simulink model "TST_EnvP_VD"  (R2016b)
settings: Solver=FixedStepDiscrete  StartTime=0.0  StopTime=simTime  FixedStep=sampleTime  RelTol=1e-3
values from neighbouring files (symbols this model uses):
  testCase = 1    [initTST_EnvP_VD_001.m]    (also in initTST_EnvP_VD_002.m = 2; initTST_EnvP_VD_003.m = 3)
libraries: simulink x7, UnitTest_Lib x3
settings Model: Creator=liangyunbo  LastModifiedBy=liangyunbo
settings DebuggingCC: SignalRangeChecking=error

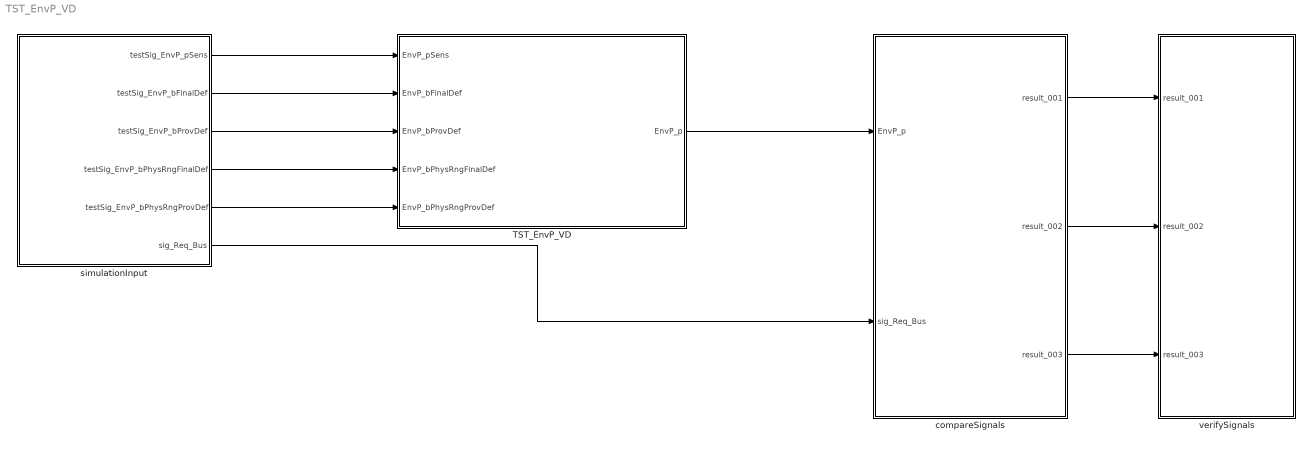
== system TST_EnvP_VD ==
  TST_EnvP_VD : Subsystem
  compareSignals : Subsystem
  simulationInput : Subsystem
  verifySignals : Subsystem
  wires:
  simulationInput/1(testSig_EnvP_pSens) -> TST_EnvP_VD/1(EnvP_pSens)
  simulationInput/2(testSig_EnvP_bFinalDef) -> TST_EnvP_VD/2(EnvP_bFinalDef)
  simulationInput/3(testSig_EnvP_bProvDef) -> TST_EnvP_VD/3(EnvP_bProvDef)
  simulationInput/4(testSig_EnvP_bPhysRngFinalDef) -> TST_EnvP_VD/4(EnvP_bPhysRngFinalDef)
  simulationInput/5(testSig_EnvP_bPhysRngProvDef) -> TST_EnvP_VD/5(EnvP_bPhysRngProvDef)
  TST_EnvP_VD/1(EnvP_p) -> compareSignals/1(EnvP_p)
  simulationInput/6(sig_Req_Bus) -> compareSignals/2(sig_Req_Bus)
  compareSignals/1(result_001) -> verifySignals/1(result_001)
  compareSignals/2(result_002) -> verifySignals/2(result_002)
  compareSignals/3(result_003) -> verifySignals/3(result_003)

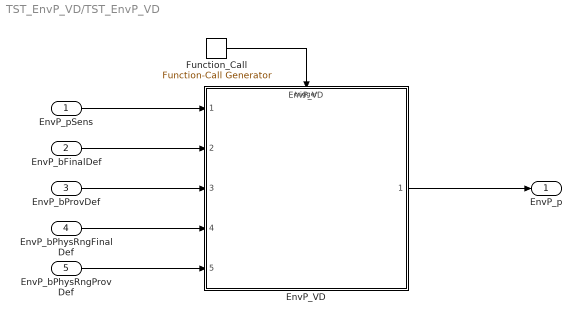
== system TST_EnvP_VD/TST_EnvP_VD ==
  EnvP_pSens : Inport
  EnvP_bFinalDef : Inport  Port=2
  EnvP_bProvDef : Inport  Port=3
  EnvP_bPhysRngFinalDef : Inport  Port=4
  EnvP_bPhysRngProvDef : Inport  Port=5
  EnvP_VD : ModelReference  ModelNameDialog=EnvP_VD  SimulationMode=Normal  ModelReferenceVersion=1.7  TriggerPortName=function  TriggerPortTriggerType=function-call  TriggerPortStatesWhenEnabling=held
  Function_Call : simulink/Ports & Subsystems/Function-Call Generator  sample_time=sampleTime  numberOfIterations=1
  EnvP_p : Outport
  wires:
  Function_Call/1 -> EnvP_VD/Trigger
  EnvP_pSens/1 -> EnvP_VD/1
  EnvP_bFinalDef/1 -> EnvP_VD/2
  EnvP_bProvDef/1 -> EnvP_VD/3
  EnvP_bPhysRngFinalDef/1 -> EnvP_VD/4
  EnvP_bPhysRngProvDef/1 -> EnvP_VD/5
  EnvP_VD/1 -> EnvP_p/1

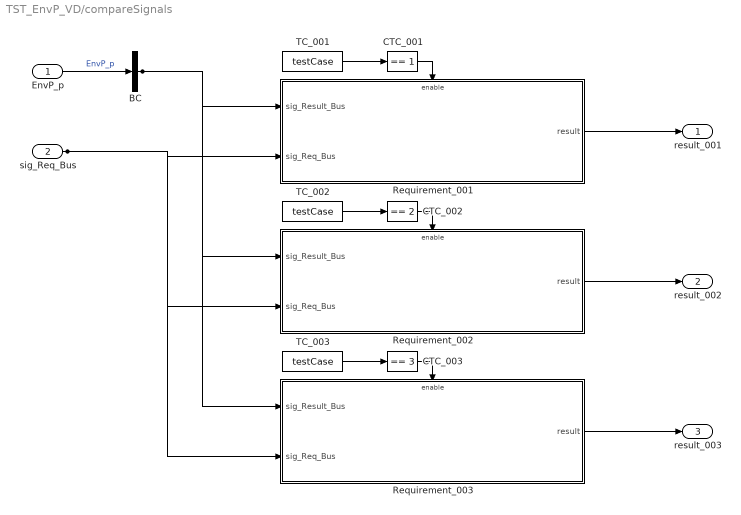
== system TST_EnvP_VD/compareSignals ==
  EnvP_p : Inport
  sig_Req_Bus : Inport  Port=2
  BC : BusCreator  Inputs=1
  CTC_001 : simulink/Logic and Bit Operations/Compare To Constant  relop===  const=1  OutDataTypeStr=boolean
  CTC_002 : simulink/Logic and Bit Operations/Compare To Constant  relop===  const=2  OutDataTypeStr=boolean
  CTC_003 : simulink/Logic and Bit Operations/Compare To Constant  relop===  const=3  OutDataTypeStr=boolean
  Requirement_001 : Subsystem
  Requirement_002 : Subsystem
  Requirement_003 : Subsystem
  TC_001 : Constant  Value=testCase
  TC_002 : Constant  Value=testCase
  TC_003 : Constant  Value=testCase
  result_001 : Outport
  result_002 : Outport  Port=2
  result_003 : Outport  Port=3
  wires:
  EnvP_p/1 -> BC/1  "EnvP_p"
  TC_001/1 -> CTC_001/1
  CTC_001/1 -> Requirement_001/Enable
  sig_Req_Bus/1 -> Requirement_001/2(sig_Req_Bus), Requirement_002/2(sig_Req_Bus), Requirement_003/2(sig_Req_Bus)
  BC/1 -> Requirement_001/1(sig_Result_Bus), Requirement_002/1(sig_Result_Bus), Requirement_003/1(sig_Result_Bus)
  Requirement_001/1(result) -> result_001/1
  TC_002/1 -> CTC_002/1
  CTC_002/1 -> Requirement_002/Enable
  Requirement_002/1(result) -> result_002/1
  TC_003/1 -> CTC_003/1
  CTC_003/1 -> Requirement_003/Enable
  Requirement_003/1(result) -> result_003/1

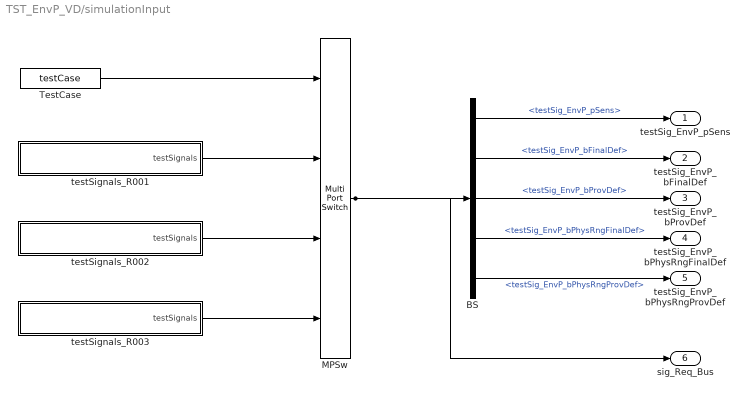
== system TST_EnvP_VD/simulationInput ==
  BS : BusSelector  OutputSignals=testSig_EnvP_pSens,testSig_EnvP_bFinalDef,testSig_EnvP_bProvDef,testSig_EnvP_bPhysRngFinalDef,testSig_EnvP_bPhysRngProvDef
  MPSw : MultiPortSwitch  SaturateOnIntegerOverflow=on  InputSameDT=on
  TestCase : Constant  Value=testCase
  testSignals_R001 : Subsystem
  testSignals_R002 : Subsystem
  testSignals_R003 : Subsystem
  testSig_EnvP_pSens : Outport
  testSig_EnvP_bFinalDef : Outport  Port=2
  testSig_EnvP_bProvDef : Outport  Port=3
  testSig_EnvP_bPhysRngFinalDef : Outport  Port=4
  testSig_EnvP_bPhysRngProvDef : Outport  Port=5
  sig_Req_Bus : Outport  Port=6
  wires:
  BS/1 -> testSig_EnvP_pSens/1  "<testSig_EnvP_pSens>"
  BS/2 -> testSig_EnvP_bFinalDef/1  "<testSig_EnvP_bFinalDef>"
  BS/3 -> testSig_EnvP_bProvDef/1  "<testSig_EnvP_bProvDef>"
  BS/4 -> testSig_EnvP_bPhysRngFinalDef/1  "<testSig_EnvP_bPhysRngFinalDef>"
  BS/5 -> testSig_EnvP_bPhysRngProvDef/1  "<testSig_EnvP_bPhysRngProvDef>"
  MPSw/1 -> BS/1, sig_Req_Bus/1
  TestCase/1 -> MPSw/1
  testSignals_R001/1(testSignals) -> MPSw/2
  testSignals_R002/1(testSignals) -> MPSw/3
  testSignals_R003/1(testSignals) -> MPSw/4

== system TST_EnvP_VD/verifySignals ==
  result_001 : Inport
  result_002 : Inport  Port=2
  result_003 : Inport  Port=3
  Assertion_001 : Assertion  Enabled=off
  Assertion_002 : Assertion  Enabled=off
  Assertion_003 : Assertion  Enabled=off
  wires:
  result_001/1 -> Assertion_001/1
  result_002/1 -> Assertion_002/1
  result_003/1 -> Assertion_003/1

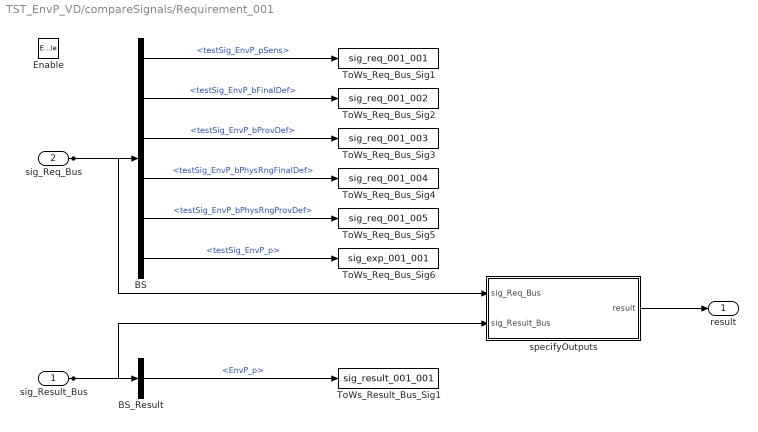
== system TST_EnvP_VD/compareSignals/Requirement_001 ==
  sig_Result_Bus : Inport
  sig_Req_Bus : Inport  Port=2
  Enable : EnablePort
  BS : BusSelector  OutputSignals=testSig_EnvP_pSens,testSig_EnvP_bFinalDef,testSig_EnvP_bProvDef,testSig_EnvP_bPhysRngFinalDef,testSig_EnvP_bPhysRngProvDef,testSig_EnvP_p
  BS_Result : BusSelector  OutputSignals=EnvP_p
  ToWs_Req_Bus_Sig1 : ToWorkspace  VariableName=sig_req_001_001  SaveFormat=Structure With Time
  ToWs_Req_Bus_Sig2 : ToWorkspace  VariableName=sig_req_001_002  SaveFormat=Structure With Time
  ToWs_Req_Bus_Sig3 : ToWorkspace  VariableName=sig_req_001_003  SaveFormat=Structure With Time
  ToWs_Req_Bus_Sig4 : ToWorkspace  VariableName=sig_req_001_004  SaveFormat=Structure With Time
  ToWs_Req_Bus_Sig5 : ToWorkspace  VariableName=sig_req_001_005  SaveFormat=Structure With Time
  ToWs_Req_Bus_Sig6 : ToWorkspace  VariableName=sig_exp_001_001  SaveFormat=Structure With Time
  ToWs_Result_Bus_Sig1 : ToWorkspace  VariableName=sig_result_001_001  SaveFormat=Structure With Time
  specifyOutputs : Subsystem
  result : Outport
  wires:
  sig_Req_Bus/1 -> BS/1, specifyOutputs/1(sig_Req_Bus)
  BS/1 -> ToWs_Req_Bus_Sig1/1  "<testSig_EnvP_pSens>"
  BS/2 -> ToWs_Req_Bus_Sig2/1  "<testSig_EnvP_bFinalDef>"
  BS/3 -> ToWs_Req_Bus_Sig3/1  "<testSig_EnvP_bProvDef>"
  BS/4 -> ToWs_Req_Bus_Sig4/1  "<testSig_EnvP_bPhysRngFinalDef>"
  BS/5 -> ToWs_Req_Bus_Sig5/1  "<testSig_EnvP_bPhysRngProvDef>"
  BS/6 -> ToWs_Req_Bus_Sig6/1  "<testSig_EnvP_p>"
  sig_Result_Bus/1 -> BS_Result/1, specifyOutputs/2(sig_Result_Bus)
  BS_Result/1 -> ToWs_Result_Bus_Sig1/1  "<EnvP_p>"
  specifyOutputs/1(result) -> result/1

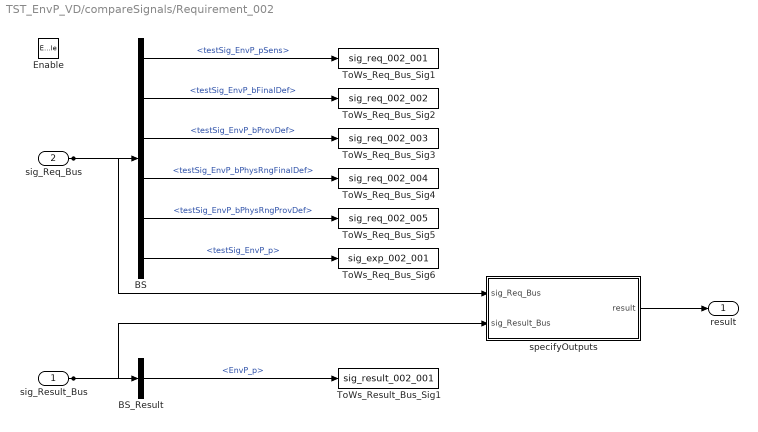
== system TST_EnvP_VD/compareSignals/Requirement_002 ==
  sig_Result_Bus : Inport
  sig_Req_Bus : Inport  Port=2
  Enable : EnablePort
  BS : BusSelector  OutputSignals=testSig_EnvP_pSens,testSig_EnvP_bFinalDef,testSig_EnvP_bProvDef,testSig_EnvP_bPhysRngFinalDef,testSig_EnvP_bPhysRngProvDef,testSig_EnvP_p
  BS_Result : BusSelector  OutputSignals=EnvP_p
  ToWs_Req_Bus_Sig1 : ToWorkspace  VariableName=sig_req_002_001  SaveFormat=Structure With Time
  ToWs_Req_Bus_Sig2 : ToWorkspace  VariableName=sig_req_002_002  SaveFormat=Structure With Time
  ToWs_Req_Bus_Sig3 : ToWorkspace  VariableName=sig_req_002_003  SaveFormat=Structure With Time
  ToWs_Req_Bus_Sig4 : ToWorkspace  VariableName=sig_req_002_004  SaveFormat=Structure With Time
  ToWs_Req_Bus_Sig5 : ToWorkspace  VariableName=sig_req_002_005  SaveFormat=Structure With Time
  ToWs_Req_Bus_Sig6 : ToWorkspace  VariableName=sig_exp_002_001  SaveFormat=Structure With Time
  ToWs_Result_Bus_Sig1 : ToWorkspace  VariableName=sig_result_002_001  SaveFormat=Structure With Time
  specifyOutputs : Subsystem
  result : Outport
  wires:
  sig_Req_Bus/1 -> BS/1, specifyOutputs/1(sig_Req_Bus)
  BS/1 -> ToWs_Req_Bus_Sig1/1  "<testSig_EnvP_pSens>"
  BS/2 -> ToWs_Req_Bus_Sig2/1  "<testSig_EnvP_bFinalDef>"
  BS/3 -> ToWs_Req_Bus_Sig3/1  "<testSig_EnvP_bProvDef>"
  BS/4 -> ToWs_Req_Bus_Sig4/1  "<testSig_EnvP_bPhysRngFinalDef>"
  BS/5 -> ToWs_Req_Bus_Sig5/1  "<testSig_EnvP_bPhysRngProvDef>"
  BS/6 -> ToWs_Req_Bus_Sig6/1  "<testSig_EnvP_p>"
  sig_Result_Bus/1 -> BS_Result/1, specifyOutputs/2(sig_Result_Bus)
  BS_Result/1 -> ToWs_Result_Bus_Sig1/1  "<EnvP_p>"
  specifyOutputs/1(result) -> result/1

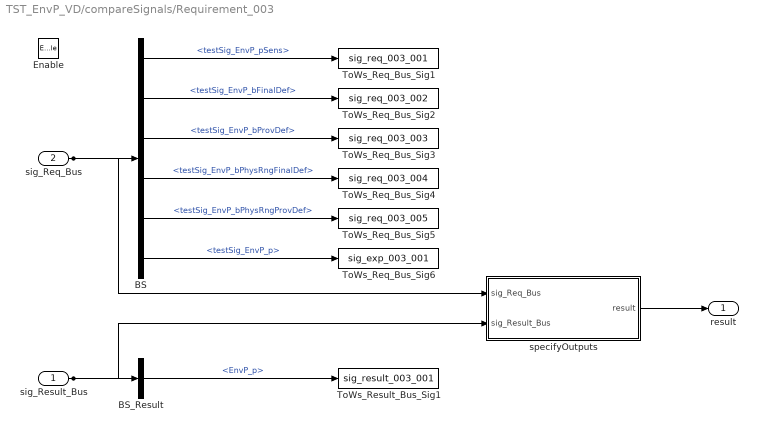
== system TST_EnvP_VD/compareSignals/Requirement_003 ==
  sig_Result_Bus : Inport
  sig_Req_Bus : Inport  Port=2
  Enable : EnablePort
  BS : BusSelector  OutputSignals=testSig_EnvP_pSens,testSig_EnvP_bFinalDef,testSig_EnvP_bProvDef,testSig_EnvP_bPhysRngFinalDef,testSig_EnvP_bPhysRngProvDef,testSig_EnvP_p
  BS_Result : BusSelector  OutputSignals=EnvP_p
  ToWs_Req_Bus_Sig1 : ToWorkspace  VariableName=sig_req_003_001  SaveFormat=Structure With Time
  ToWs_Req_Bus_Sig2 : ToWorkspace  VariableName=sig_req_003_002  SaveFormat=Structure With Time
  ToWs_Req_Bus_Sig3 : ToWorkspace  VariableName=sig_req_003_003  SaveFormat=Structure With Time
  ToWs_Req_Bus_Sig4 : ToWorkspace  VariableName=sig_req_003_004  SaveFormat=Structure With Time
  ToWs_Req_Bus_Sig5 : ToWorkspace  VariableName=sig_req_003_005  SaveFormat=Structure With Time
  ToWs_Req_Bus_Sig6 : ToWorkspace  VariableName=sig_exp_003_001  SaveFormat=Structure With Time
  ToWs_Result_Bus_Sig1 : ToWorkspace  VariableName=sig_result_003_001  SaveFormat=Structure With Time
  specifyOutputs : Subsystem
  result : Outport
  wires:
  sig_Req_Bus/1 -> BS/1, specifyOutputs/1(sig_Req_Bus)
  BS/1 -> ToWs_Req_Bus_Sig1/1  "<testSig_EnvP_pSens>"
  BS/2 -> ToWs_Req_Bus_Sig2/1  "<testSig_EnvP_bFinalDef>"
  BS/3 -> ToWs_Req_Bus_Sig3/1  "<testSig_EnvP_bProvDef>"
  BS/4 -> ToWs_Req_Bus_Sig4/1  "<testSig_EnvP_bPhysRngFinalDef>"
  BS/5 -> ToWs_Req_Bus_Sig5/1  "<testSig_EnvP_bPhysRngProvDef>"
  BS/6 -> ToWs_Req_Bus_Sig6/1  "<testSig_EnvP_p>"
  sig_Result_Bus/1 -> BS_Result/1, specifyOutputs/2(sig_Result_Bus)
  BS_Result/1 -> ToWs_Result_Bus_Sig1/1  "<EnvP_p>"
  specifyOutputs/1(result) -> result/1

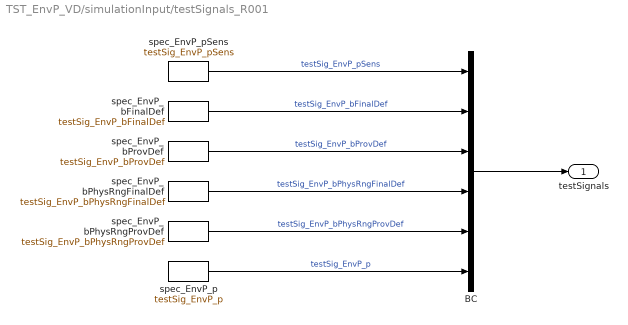
== system TST_EnvP_VD/simulationInput/testSignals_R001 ==
  BC : BusCreator  Inputs=6
  spec_EnvP_bFinalDef : FromWorkspace  VariableName=testSig_EnvP_bFinalDef  Interpolate=off  OutputAfterFinalValue=Holding final value
  spec_EnvP_bPhysRngFinalDef : FromWorkspace  VariableName=testSig_EnvP_bPhysRngFinalDef  Interpolate=off  OutputAfterFinalValue=Holding final value
  spec_EnvP_bPhysRngProvDef : FromWorkspace  VariableName=testSig_EnvP_bPhysRngProvDef  Interpolate=off  OutputAfterFinalValue=Holding final value
  spec_EnvP_bProvDef : FromWorkspace  VariableName=testSig_EnvP_bProvDef  Interpolate=off  OutputAfterFinalValue=Holding final value
  spec_EnvP_p : FromWorkspace  VariableName=testSig_EnvP_p  Interpolate=off  OutputAfterFinalValue=Holding final value
  spec_EnvP_pSens : FromWorkspace  VariableName=testSig_EnvP_pSens  Interpolate=off  OutputAfterFinalValue=Holding final value
  testSignals : Outport
  wires:
  BC/1 -> testSignals/1
  spec_EnvP_pSens/1 -> BC/1  "testSig_EnvP_pSens"
  spec_EnvP_bFinalDef/1 -> BC/2  "testSig_EnvP_bFinalDef"
  spec_EnvP_bProvDef/1 -> BC/3  "testSig_EnvP_bProvDef"
  spec_EnvP_bPhysRngFinalDef/1 -> BC/4  "testSig_EnvP_bPhysRngFinalDef"
  spec_EnvP_bPhysRngProvDef/1 -> BC/5  "testSig_EnvP_bPhysRngProvDef"
  spec_EnvP_p/1 -> BC/6  "testSig_EnvP_p"

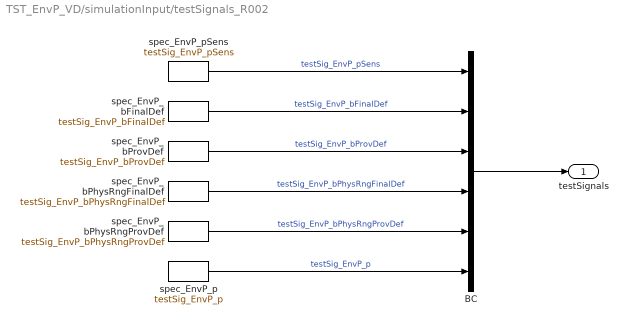
== system TST_EnvP_VD/simulationInput/testSignals_R002 ==
  BC : BusCreator  Inputs=6
  spec_EnvP_bFinalDef : FromWorkspace  VariableName=testSig_EnvP_bFinalDef  Interpolate=off  OutputAfterFinalValue=Holding final value
  spec_EnvP_bPhysRngFinalDef : FromWorkspace  VariableName=testSig_EnvP_bPhysRngFinalDef  Interpolate=off  OutputAfterFinalValue=Holding final value
  spec_EnvP_bPhysRngProvDef : FromWorkspace  VariableName=testSig_EnvP_bPhysRngProvDef  Interpolate=off  OutputAfterFinalValue=Holding final value
  spec_EnvP_bProvDef : FromWorkspace  VariableName=testSig_EnvP_bProvDef  Interpolate=off  OutputAfterFinalValue=Holding final value
  spec_EnvP_p : FromWorkspace  VariableName=testSig_EnvP_p  Interpolate=off  OutputAfterFinalValue=Holding final value
  spec_EnvP_pSens : FromWorkspace  VariableName=testSig_EnvP_pSens  Interpolate=off  OutputAfterFinalValue=Holding final value
  testSignals : Outport
  wires:
  BC/1 -> testSignals/1
  spec_EnvP_pSens/1 -> BC/1  "testSig_EnvP_pSens"
  spec_EnvP_bFinalDef/1 -> BC/2  "testSig_EnvP_bFinalDef"
  spec_EnvP_bProvDef/1 -> BC/3  "testSig_EnvP_bProvDef"
  spec_EnvP_bPhysRngFinalDef/1 -> BC/4  "testSig_EnvP_bPhysRngFinalDef"
  spec_EnvP_bPhysRngProvDef/1 -> BC/5  "testSig_EnvP_bPhysRngProvDef"
  spec_EnvP_p/1 -> BC/6  "testSig_EnvP_p"

== system TST_EnvP_VD/simulationInput/testSignals_R003 ==
  BC : BusCreator  Inputs=6
  spec_EnvP_bFinalDef : FromWorkspace  VariableName=testSig_EnvP_bFinalDef  Interpolate=off  OutputAfterFinalValue=Holding final value
  spec_EnvP_bPhysRngFinalDef : FromWorkspace  VariableName=testSig_EnvP_bPhysRngFinalDef  Interpolate=off  OutputAfterFinalValue=Holding final value
  spec_EnvP_bPhysRngProvDef : FromWorkspace  VariableName=testSig_EnvP_bPhysRngProvDef  Interpolate=off  OutputAfterFinalValue=Holding final value
  spec_EnvP_bProvDef : FromWorkspace  VariableName=testSig_EnvP_bProvDef  Interpolate=off  OutputAfterFinalValue=Holding final value
  spec_EnvP_p : FromWorkspace  VariableName=testSig_EnvP_p  Interpolate=off  OutputAfterFinalValue=Holding final value
  spec_EnvP_pSens : FromWorkspace  VariableName=testSig_EnvP_pSens  Interpolate=off  OutputAfterFinalValue=Holding final value
  testSignals : Outport
  wires:
  BC/1 -> testSignals/1
  spec_EnvP_pSens/1 -> BC/1  "testSig_EnvP_pSens"
  spec_EnvP_bFinalDef/1 -> BC/2  "testSig_EnvP_bFinalDef"
  spec_EnvP_bProvDef/1 -> BC/3  "testSig_EnvP_bProvDef"
  spec_EnvP_bPhysRngFinalDef/1 -> BC/4  "testSig_EnvP_bPhysRngFinalDef"
  spec_EnvP_bPhysRngProvDef/1 -> BC/5  "testSig_EnvP_bPhysRngProvDef"
  spec_EnvP_p/1 -> BC/6  "testSig_EnvP_p"

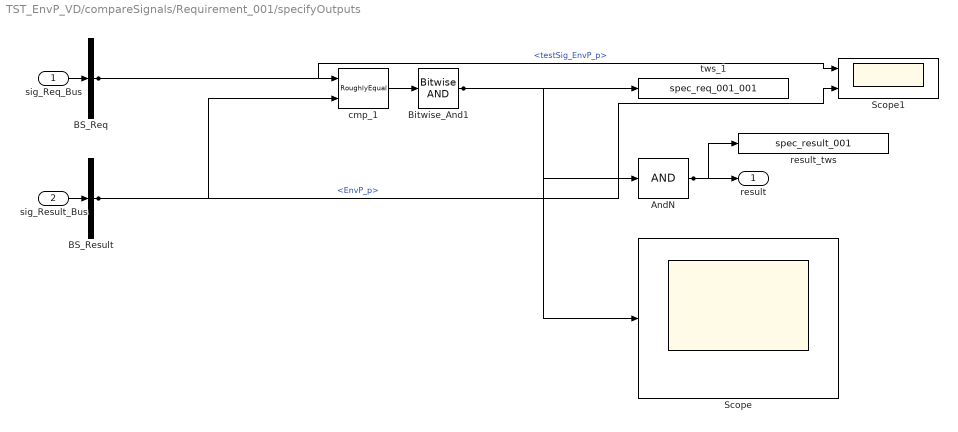
== system TST_EnvP_VD/compareSignals/Requirement_001/specifyOutputs ==
  sig_Req_Bus : Inport
  sig_Result_Bus : Inport  Port=2
  AndN : Logic  Inputs=1
  BS_Req : BusSelector  OutputSignals=testSig_EnvP_p
  BS_Result : BusSelector  OutputSignals=EnvP_p
  Bitwise_And1 : simulink/Logic and Bit Operations/Bitwise Operator  logicop=AND  UseBitMask=off  BitMask=bin2dec('11011001')  BitMaskRealWorld=Stored Integer
  Scope : Scope
  Scope1 : Scope  NumInputPorts=2
  cmp_1 : UnitTest_Lib/RoughlyEqual  slope=0.1
  result_tws : ToWorkspace  VariableName=spec_result_001
  tws_1 : ToWorkspace  VariableName=spec_req_001_001
  result : Outport
  wires:
  sig_Req_Bus/1 -> BS_Req/1
  sig_Result_Bus/1 -> BS_Result/1
  AndN/1 -> result/1, result_tws/1
  BS_Req/1 -> cmp_1/1, Scope1/1  "<testSig_EnvP_p>"
  BS_Result/1 -> cmp_1/2, Scope1/2  "<EnvP_p>"
  cmp_1/1 -> Bitwise_And1/1
  Bitwise_And1/1 -> tws_1/1, AndN/1, Scope/1

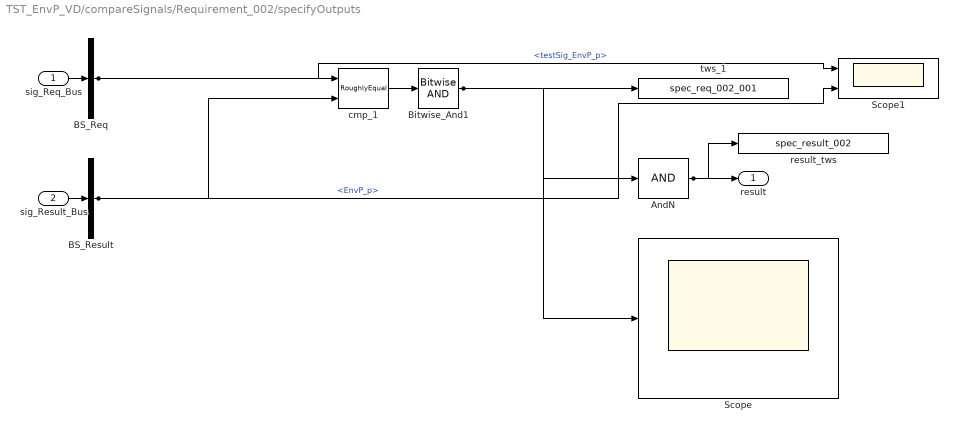
== system TST_EnvP_VD/compareSignals/Requirement_002/specifyOutputs ==
  sig_Req_Bus : Inport
  sig_Result_Bus : Inport  Port=2
  AndN : Logic  Inputs=1
  BS_Req : BusSelector  OutputSignals=testSig_EnvP_p
  BS_Result : BusSelector  OutputSignals=EnvP_p
  Bitwise_And1 : simulink/Logic and Bit Operations/Bitwise Operator  logicop=AND  UseBitMask=off  BitMask=bin2dec('11011001')  BitMaskRealWorld=Stored Integer
  Scope : Scope
  Scope1 : Scope  NumInputPorts=2
  cmp_1 : UnitTest_Lib/RoughlyEqual  slope=0.1
  result_tws : ToWorkspace  VariableName=spec_result_002
  tws_1 : ToWorkspace  VariableName=spec_req_002_001
  result : Outport
  wires:
  sig_Req_Bus/1 -> BS_Req/1
  sig_Result_Bus/1 -> BS_Result/1
  AndN/1 -> result/1, result_tws/1
  BS_Req/1 -> cmp_1/1, Scope1/1  "<testSig_EnvP_p>"
  BS_Result/1 -> cmp_1/2, Scope1/2  "<EnvP_p>"
  cmp_1/1 -> Bitwise_And1/1
  Bitwise_And1/1 -> tws_1/1, AndN/1, Scope/1

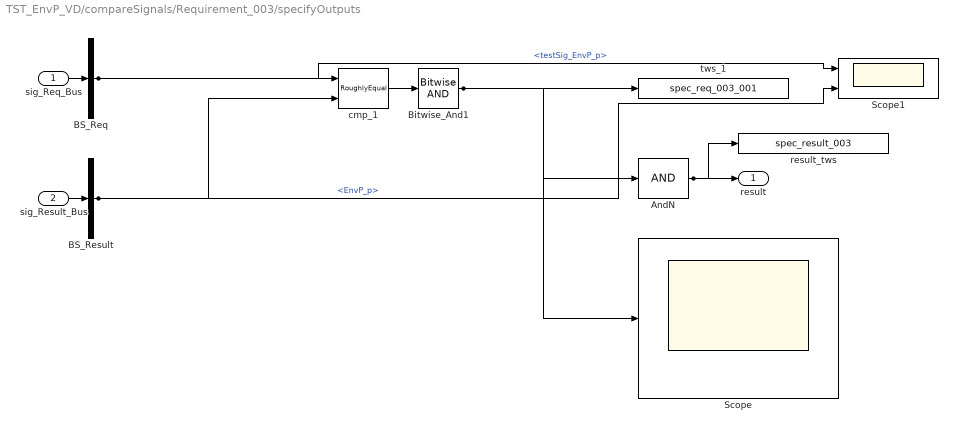
== system TST_EnvP_VD/compareSignals/Requirement_003/specifyOutputs ==
  sig_Req_Bus : Inport
  sig_Result_Bus : Inport  Port=2
  AndN : Logic  Inputs=1
  BS_Req : BusSelector  OutputSignals=testSig_EnvP_p
  BS_Result : BusSelector  OutputSignals=EnvP_p
  Bitwise_And1 : simulink/Logic and Bit Operations/Bitwise Operator  logicop=AND  UseBitMask=off  BitMask=bin2dec('11011001')  BitMaskRealWorld=Stored Integer
  Scope : Scope
  Scope1 : Scope  NumInputPorts=2
  cmp_1 : UnitTest_Lib/RoughlyEqual  slope=0.1
  result_tws : ToWorkspace  VariableName=spec_result_003
  tws_1 : ToWorkspace  VariableName=spec_req_003_001
  result : Outport
  wires:
  sig_Req_Bus/1 -> BS_Req/1
  sig_Result_Bus/1 -> BS_Result/1
  AndN/1 -> result/1, result_tws/1
  BS_Req/1 -> cmp_1/1, Scope1/1  "<testSig_EnvP_p>"
  BS_Result/1 -> cmp_1/2, Scope1/2  "<EnvP_p>"
  cmp_1/1 -> Bitwise_And1/1
  Bitwise_And1/1 -> tws_1/1, AndN/1, Scope/1
